simulink model "Parabolic_sim"  (R2017a)
settings: Solver=VariableStepAuto  StartTime=0.0  StopTime=50  RelTol=1e-3
values from neighbouring files (symbols this model uses):
  b = 2.8956    [Aerosonde_coeff.m]    (also in coeff_Aerosonde.m)
  c = 0.18994    [Aerosonde_coeff.m]    (also in coeff_Aerosonde.m)
  C_De = 0    [Aerosonde_coeff.m]    (also in coeff_Aerosonde.m)
  C_Dq = 0    [Aerosonde_coeff.m]    (also in coeff_Aerosonde.m)
  C_Le = -0.36    [Aerosonde_coeff.m]    (also in coeff_Aerosonde.m)
  C_Lq = 0    [Aerosonde_coeff.m]    (also in coeff_Aerosonde.m)
  C_m0 = -0.02338    [Aerosonde_coeff.m]    (also in coeff_Aerosonde.m)
  C_ma = -0.38    [Aerosonde_coeff.m]    (also in coeff_Aerosonde.m)
  C_me = -0.5    [Aerosonde_coeff.m]    (also in coeff_Aerosonde.m)
  C_mq = -3.6    [Aerosonde_coeff.m]    (also in coeff_Aerosonde.m)
  rho = 1.2682    [Aerosonde_coeff.m]    (also in coeff_Aerosonde.m)
undefined symbols (not defined in the file or in its folder): Newton, Raphson, sigbuilder_block
libraries: simulink_extras x7, aerolibasang x3, shared3dof x1, aerolibadyn x1
settings Model: Creator=jljoberg  LastModifiedBy=jljoberg

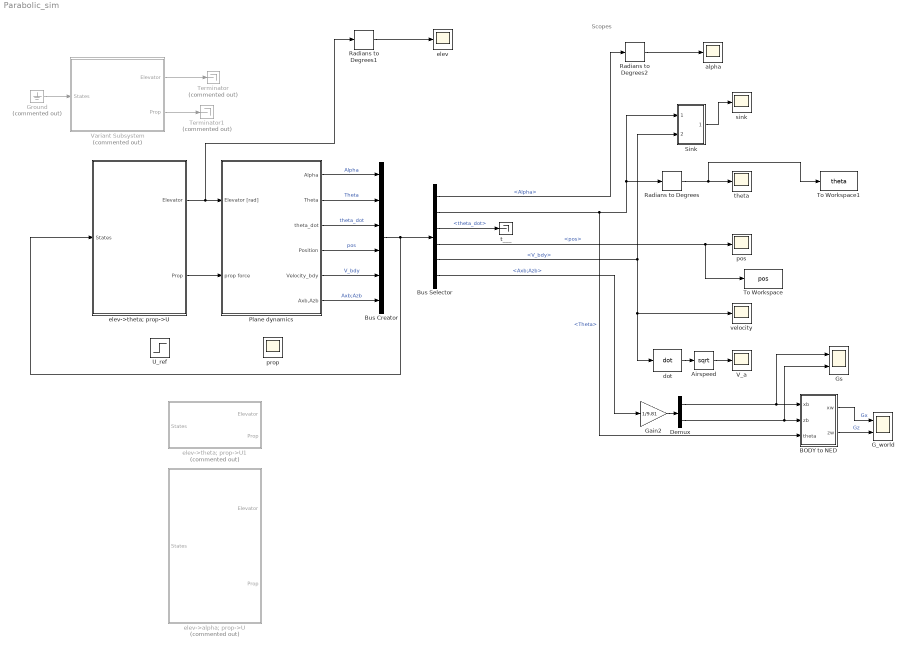
== system Parabolic_sim ==
  note: Scopes
  Airspeed : Sqrt  AlgorithmType=Newton-Raphson  SaturateOnIntegerOverflow=on
  BODY to NED : Subsystem
  Bus Creator : BusCreator  Inputs=6
  Bus Selector : BusSelector  OutputSignals=Alpha,Theta,theta_dot,pos,V_bdy,Axb;Azb
  Demux : Demux  Outputs=2
  G_world : Scope  NumInputPorts=2
  Gain2 : Gain  Gain=1/9.81
  Ground : Ground  Commented=on
  Gs : Scope  NumInputPorts=2
  Plane dynamics : Subsystem
  Radians to Degrees : simulink_extras/Transformations/Radians to Degrees
  Radians to Degrees1 : simulink_extras/Transformations/Radians to Degrees
  Radians to Degrees2 : simulink_extras/Transformations/Radians to Degrees
  Sink : Subsystem
  Terminator : Terminator  Commented=on
  Terminator1 : Terminator  Commented=on
  To Workspace : ToWorkspace  VariableName=pos  SaveFormat=Timeseries  SampleTime=-1
  To Workspace1 : ToWorkspace  VariableName=theta  SaveFormat=Timeseries  SampleTime=-1
  U_ref : Step  Time=10.5  Before=10  After=5  SampleTime=0
  V_a : Scope
  Variant Subsystem : Subsystem  Commented=on  Variant=on  OverrideUsingVariant=(default)
  alpha : Scope
  dot : aerolibasang/Incidence  & Airspeed/dot
      settings: SourceProductName=Aerospace Blockset  SourceProductBaseCode=AE
  elev : Scope
  elev->alpha; prop->U : Subsystem  Commented=on  VariantControl=Variant
  elev->theta; prop->U : Subsystem  VariantControl=Variant
  elev->theta; prop->U1 : Subsystem  Commented=on  VariantControl=(default)
  pos : Scope
  prop : Scope
  sink : Scope
  t___ : Terminator
  theta : Scope
  velocity : Scope
  wires:
  Bus Selector/1 -> Radians to Degrees2/1  "<Alpha>"
  Bus Selector/2 -> BODY to NED/3(theta), Radians to Degrees/1, Sink/1(theta)  "<Theta>"
  Bus Selector/3 -> t___/1  "<theta_dot>"
  Bus Selector/4 -> To Workspace/1, pos/1  "<pos>"
  Bus Selector/5 -> dot/1, velocity/1, Sink/2(v_bdy)  "<V_bdy>"
  Airspeed/1 -> V_a/1
  dot/1 -> Airspeed/1
  Radians to Degrees/1 -> To Workspace1/1, theta/1
  Sink/1(sink) -> sink/1
  Plane dynamics/6(Axb,Azb) -> Bus Creator/6  "Axb;Azb"
  Plane dynamics/5(Velocity_bdy) -> Bus Creator/5  "V_bdy"
  Plane dynamics/4(Position) -> Bus Creator/4  "pos"
  Plane dynamics/3(theta_dot) -> Bus Creator/3  "theta_dot"
  Plane dynamics/2(Theta) -> Bus Creator/2  "Theta"
  Plane dynamics/1(Alpha) -> Bus Creator/1  "Alpha"
  Bus Creator/1 -> elev->theta; prop->U/1(States), Bus Selector/1
  Radians to Degrees2/1 -> alpha/1
  Ground/1 -> Variant Subsystem/1(States)
  Variant Subsystem/1(Elevator) -> Terminator/1
  Variant Subsystem/2(Prop) -> Terminator1/1
  Bus Selector/6 -> Gain2/1  "<Axb;Azb>"
  Radians to Degrees1/1 -> elev/1
  elev->theta; prop->U/1(Elevator) -> Radians to Degrees1/1, Plane dynamics/1(Elevator [rad])
  Gain2/1 -> Demux/1
  Demux/1 -> BODY to NED/1(xb), Gs/1
  Demux/2 -> BODY to NED/2(zb), Gs/2
  BODY to NED/1(xw) -> G_world/1  "Gx"
  BODY to NED/2(zw) -> G_world/2  "Gz"
  elev->theta; prop->U/2(Prop) -> Plane dynamics/2(prop force)

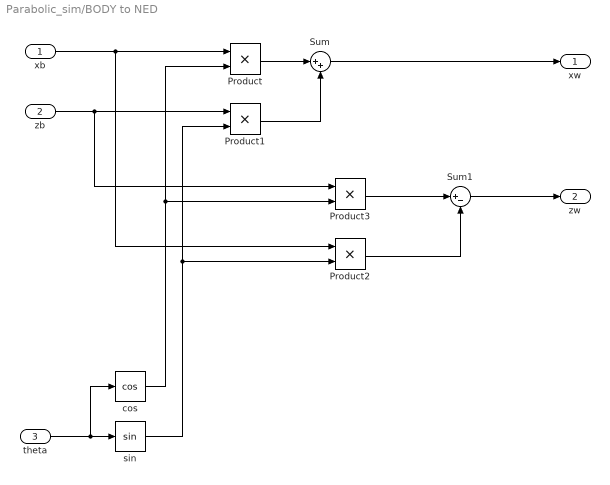
== system Parabolic_sim/BODY to NED ==
  xb : Inport
  zb : Inport  Port=2
  theta : Inport  Port=3
  Product{,1..3} (4 alike) : Product
  Sum : Sum  Inputs=|++
  Sum1 : Sum  Inputs=|+-
  "cos " : Trigonometry  Operator=cos
  sin : Trigonometry
  xw : Outport
  zw : Outport  Port=2
  wires:
  theta/1 -> sin/1, "cos "/1
  xb/1 -> Product/1, Product2/1
  "cos "/1 -> Product3/2, Product/2
  Product/1 -> Sum/1
  Sum/1 -> xw/1
  zb/1 -> Product3/1, Product1/1
  sin/1 -> Product1/2, Product2/2
  Product1/1 -> Sum/2
  Sum1/1 -> zw/1
  Product3/1 -> Sum1/1
  Product2/1 -> Sum1/2

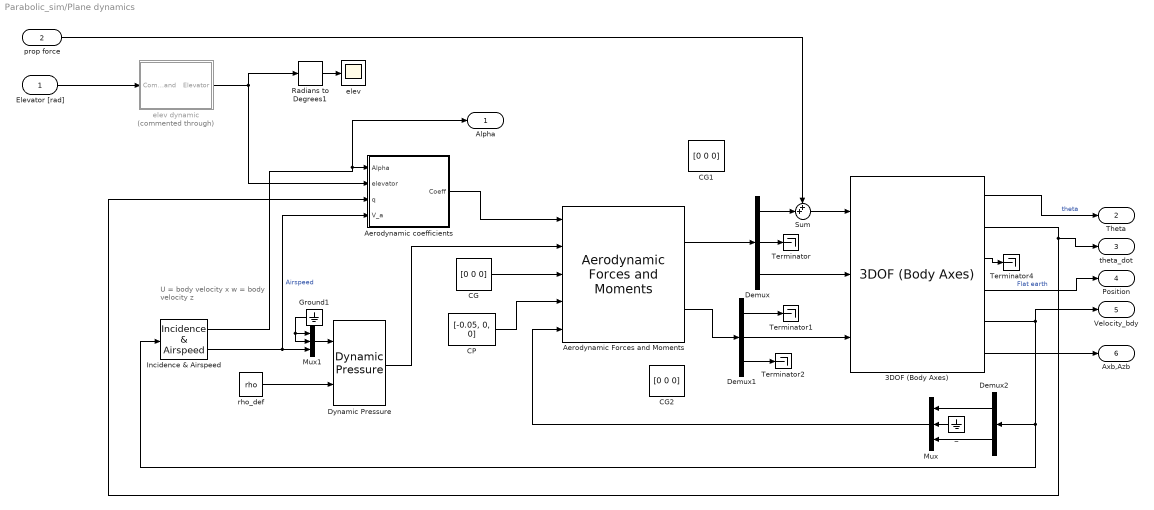
== system Parabolic_sim/Plane dynamics ==
  note: U = body velocity x
      | w = body velocity z
  Elevator [rad] : Inport
  prop force : Inport  Port=2
  3DOF (Body Axes) : shared3dof/3DOF (Body Axes)  units=Metric (MKS)  mtype=Fixed  v_ini=30  theta_ini=60*deg2rad  alpha_ini=0  q_ini=0*deg2rad  pos_ini=[0 0]  mass=m  mass_e=0.5  mass_f=3.0  Iyy=Jy  Iyy_e=0.5  Iyy_f=3.0  g_in=Internal  g=9.81  vre_flag=on  abi_flag=off
  "Aerodynamic Forces and Moments " : aerolibadyn/Aerodynamic Forces and Moments   inputAxes=Wind  outputForceAxes=Body  outputMomentAxes=Wind  S=S  b=b  cbar=1
      settings: SourceProductName=Aerospace Blockset
  Aerodynamic coefficients : Subsystem
  CG : Constant  Value=[0 0 0]
  CG1 : Constant  Value=[0 0 0]
  CG2 : Constant  Value=[0 0 0]
  CP : Constant  Value=[-0.05, 0, 0]
  Demux : Demux  Outputs=3
  Demux1 : Demux  Outputs=3
  Demux2 : Demux  Outputs=2
  Dynamic Pressure : aerolibasang/Dynamic Pressure
  Ground1 : Ground
  Incidence & Airspeed : aerolibasang/Incidence  & Airspeed
      settings: SourceProductName=Aerospace Blockset  SourceProductBaseCode=AE
  Mux : Mux  Inputs=3
  Mux1 : Mux  Inputs=3
  Radians to Degrees1 : simulink_extras/Transformations/Radians to Degrees
  Sum : Sum  Inputs=++|
  Terminator{,1..2,4} (4 alike) : Terminator
  _ : Ground
  elev : Scope
  elev dynamic : Subsystem  Commented=through
  rho_def : Constant  Value=rho
  Alpha : Outport
  Theta : Outport  Port=2
  theta_dot : Outport  Port=3
  Position : Outport  Port=4
  Velocity_bdy : Outport  Port=5
  Axb,Azb : Outport  Port=6
  wires:
  Ground1/1 -> Mux1/1, Mux1/2
  3DOF (Body Axes)/2 -> Aerodynamic coefficients/3(q), theta_dot/1
  3DOF (Body Axes)/3 -> Terminator4/1
  Incidence & Airspeed/1 -> Alpha/1, Aerodynamic coefficients/1(Alpha)
  rho_def/1 -> Dynamic Pressure/2
  Aerodynamic coefficients/1(Coeff) -> "Aerodynamic Forces and Moments "/1
  Incidence & Airspeed/2 -> Mux1/3, Aerodynamic coefficients/4(V_a)  "Airspeed"
  3DOF (Body Axes)/5 -> Velocity_bdy/1, Incidence & Airspeed/1, Demux2/1
  Dynamic Pressure/1 -> "Aerodynamic Forces and Moments "/2
  Demux/3 -> 3DOF (Body Axes)/2
  3DOF (Body Axes)/1 -> Theta/1  "theta"
  3DOF (Body Axes)/6 -> Axb,Azb/1
  Demux/2 -> Terminator/1
  3DOF (Body Axes)/4 -> Position/1  "Flat earth"
  CG/1 -> "Aerodynamic Forces and Moments "/3
  CP/1 -> "Aerodynamic Forces and Moments "/4
  Demux2/1 -> Mux/1
  Demux1/2 -> 3DOF (Body Axes)/3
  _/1 -> Mux/2
  Demux1/1 -> Terminator1/1
  Demux1/3 -> Terminator2/1
  Demux2/2 -> Mux/3
  Mux/1 -> "Aerodynamic Forces and Moments "/5
  Mux1/1 -> Dynamic Pressure/1
  Sum/1 -> 3DOF (Body Axes)/1
  prop force/1 -> Sum/1
  Demux/1 -> Sum/2
  Radians to Degrees1/1 -> elev/1
  Elevator [rad]/1 -> elev dynamic/1(Command)
  elev dynamic/1(Elevator) -> Aerodynamic coefficients/2(elevator), Radians to Degrees1/1
  "Aerodynamic Forces and Moments "/2 -> Demux1/1
  "Aerodynamic Forces and Moments "/1 -> Demux/1

== system Parabolic_sim/Sink ==
  theta : Inport
  v_bdy : Inport  Port=2
  Demux : Demux  Outputs=2
  Product : Product
  Product1 : Product
  Sum : Sum  Inputs=-+|
  Trigonometric Function : Trigonometry  Operator=cos
  Trigonometric Function1 : Trigonometry
  sink : Outport
  wires:
  v_bdy/1 -> Demux/1
  theta/1 -> Trigonometric Function1/1, Trigonometric Function/1
  Product/1 -> Sum/2
  Product1/1 -> Sum/1
  Sum/1 -> sink/1
  Trigonometric Function/1 -> Product/2
  Demux/2 -> Product/1
  Demux/1 -> Product1/2
  Trigonometric Function1/1 -> Product1/1

== system Parabolic_sim/Variant Subsystem ==
  note: 1) Add Subsystem or Model blocks as valid variant choices.
      | 2) You cannot connect blocks at this level. At simulation, connectivity is automatically
      | determined, based on the active variant and port name matching.
  States : Inport
  elev->theta; prop->U : Subsystem  VariantControl=(default)
  Elevator : Outport
  Prop : Outport  Port=2

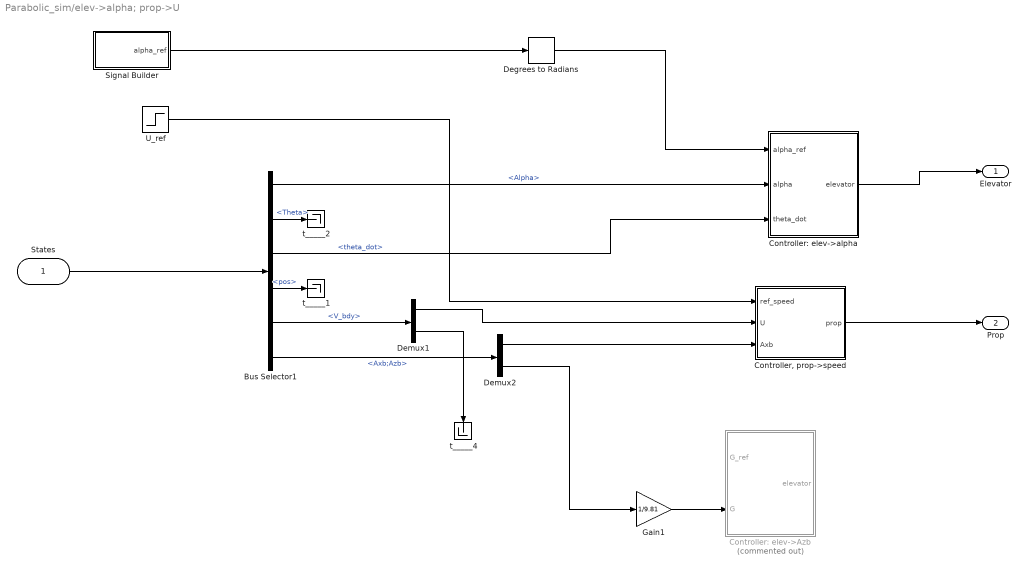
== system Parabolic_sim/elev->alpha; prop->U ==
  States : Inport
  Bus Selector1 : BusSelector  OutputSignals=Alpha,Theta,theta_dot,pos,V_bdy,Axb;Azb
  "Controller, prop->speed" : Subsystem
  Controller: elev->Azb : Subsystem  Commented=on
  Controller: elev->alpha : Subsystem
  Degrees to Radians : simulink_extras/Transformations/Degrees to Radians
  Demux1 : Demux  Outputs=2
  Demux2 : Demux  Outputs=2
  Gain1 : Gain  Gain=1/9.81
  Signal Builder : Subsystem  Tag=STV Subsys  LoadFcn=sigbuilder_block('load');  StartFcn=sigbuilder_block('start');  StopFcn=sigbuilder_block('stop');  ClipboardFcn=sigbuilder_block('clipboard');  mask(Sigbuilder block){tuvar=[0:10]}
      mask help: Simulink:masks:SigbuilderBlock_MD
      mask init:
      | if ~strcmp(get_param(bdroot(gcbh),'SimulationStatus'),'stopped') tuvar = sigbuilder_block('maskInit'); end
      settings: CopyFcn=sigbuilder_block('copy');  DeleteFcn=sigbuilder_block('delete');  ModelCloseFcn=sigbuilder_block('modelClose');  PreSaveFcn=sigbuilder_block('preSave');  PauseFcn=sigbuilder_block('pause');  ContinueFcn=sigbuilder_block('continue');  NameChangeFcn=sigbuilder_block('namechange');  OpenFcn=sigbuilder_block('open',[254.25 194.25 787.5 402 ]);  CloseFcn=sigbuilder_block('close');
      mask Display: plot(0, 0, 100, 100,[2, 2, 32, 32, 2], [68, 8, 8, 68, 68],[32, 2], [38, 38], [32, 19, 2],[53, 60, 44], [32, 17, 17, 2],[16, 16, 31, 31]);txt = getActiveGroup(gcbh);text(2, 100, txt,'verticalAlignment', 'top');
  U_ref : Step  Time=150  Before=25  After=25  SampleTime=0
  t_____1 : Terminator
  t_____2 : Terminator
  t_____4 : Terminator
  Elevator : Outport
  Prop : Outport  Port=2
  wires:
  "Controller, prop->speed"/1(prop) -> Prop/1
  Demux1/1 -> "Controller, prop->speed"/2(U)
  Demux2/2 -> Gain1/1
  Bus Selector1/5 -> Demux1/1  "<V_bdy>"
  Bus Selector1/6 -> Demux2/1  "<Axb;Azb>"
  Demux2/1 -> "Controller, prop->speed"/3(Axb)
  States/1 -> Bus Selector1/1
  Demux1/2 -> t_____4/1
  Bus Selector1/4 -> t_____1/1  "<pos>"
  Gain1/1 -> Controller: elev->Azb/2(G)
  Controller: elev->alpha/1(elevator) -> Elevator/1
  Bus Selector1/1 -> Controller: elev->alpha/2(alpha)  "<Alpha>"
  U_ref/1 -> "Controller, prop->speed"/1(ref_speed)
  Signal Builder/1(alpha_ref) -> Degrees to Radians/1
  Degrees to Radians/1 -> Controller: elev->alpha/1(alpha_ref)
  Bus Selector1/2 -> t_____2/1  "<Theta>"
  Bus Selector1/3 -> Controller: elev->alpha/3(theta_dot)  "<theta_dot>"

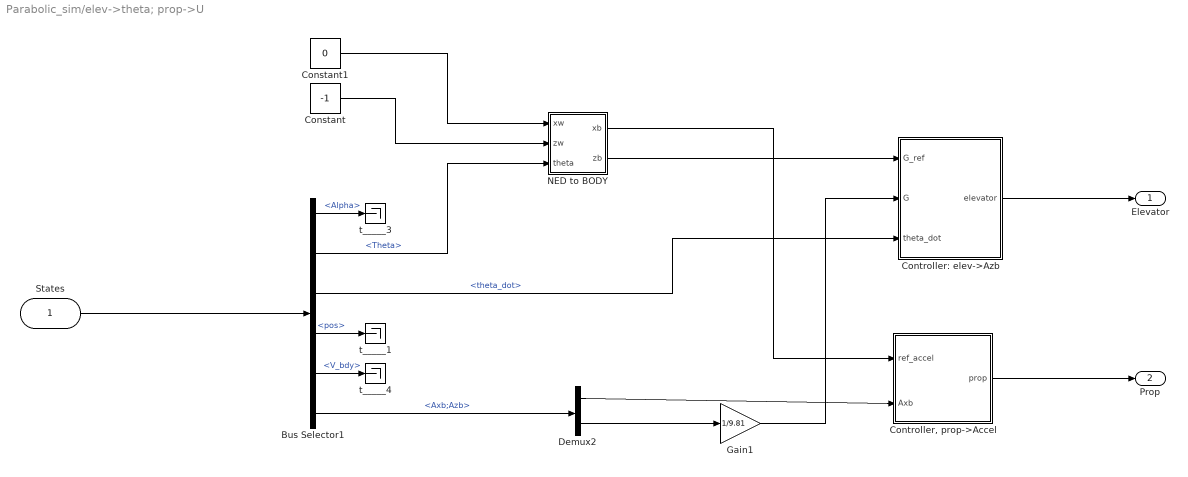
== system Parabolic_sim/elev->theta; prop->U ==
  States : Inport
  Bus Selector1 : BusSelector  OutputSignals=Alpha,Theta,theta_dot,pos,V_bdy,Axb;Azb
  Constant : Constant  Value=-1
  Constant1 : Constant  Value=0
  "Controller, prop->Accel" : Subsystem
  Controller: elev->Azb : Subsystem
  Demux2 : Demux  Outputs=2
  Gain1 : Gain  Gain=1/9.81
  NED to BODY : Subsystem
  t_____1 : Terminator
  t_____3 : Terminator
  t_____4 : Terminator
  Elevator : Outport
  Prop : Outport  Port=2
  wires:
  "Controller, prop->Accel"/1(prop) -> Prop/1
  Demux2/2 -> Gain1/1
  Bus Selector1/6 -> Demux2/1  "<Axb;Azb>"
  Demux2/1 -> "Controller, prop->Accel"/2(Axb)
  States/1 -> Bus Selector1/1
  Bus Selector1/4 -> t_____1/1  "<pos>"
  Gain1/1 -> Controller: elev->Azb/2(G)
  Controller: elev->Azb/1(elevator) -> Elevator/1
  Bus Selector1/1 -> t_____3/1  "<Alpha>"
  Bus Selector1/2 -> NED to BODY/3(theta)  "<Theta>"
  Bus Selector1/3 -> Controller: elev->Azb/3(theta_dot)  "<theta_dot>"
  Constant/1 -> NED to BODY/2(zw)
  Constant1/1 -> NED to BODY/1(xw)
  NED to BODY/2(zb) -> Controller: elev->Azb/1(G_ref)
  NED to BODY/1(xb) -> "Controller, prop->Accel"/1(ref_accel)
  Bus Selector1/5 -> t_____4/1  "<V_bdy>"

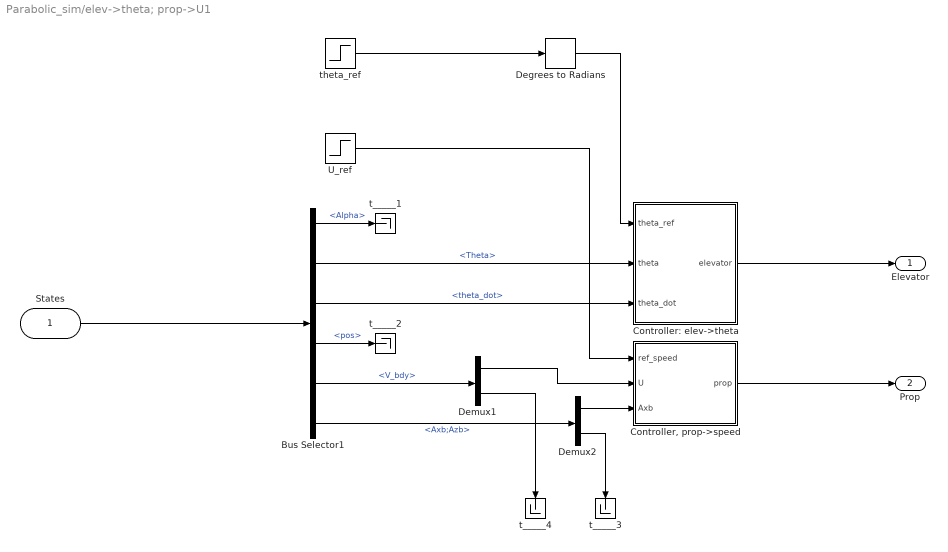
== system Parabolic_sim/elev->theta; prop->U1 ==
  States : Inport
  Bus Selector1 : BusSelector  OutputSignals=Alpha,Theta,theta_dot,pos,V_bdy,Axb;Azb
  "Controller, prop->speed" : Subsystem
  Controller: elev->theta : Subsystem
  Degrees to Radians : simulink_extras/Transformations/Degrees to Radians
  Demux1 : Demux  Outputs=2
  Demux2 : Demux  Outputs=2
  U_ref : Step  Time=150  Before=20  After=30  SampleTime=0
  t_____{1..4} (4 alike) : Terminator
  theta_ref : Step  Time=180  After=30  SampleTime=0
  Elevator : Outport
  Prop : Outport  Port=2
  wires:
  theta_ref/1 -> Degrees to Radians/1
  Degrees to Radians/1 -> Controller: elev->theta/1(theta_ref)
  Controller: elev->theta/1(elevator) -> Elevator/1
  "Controller, prop->speed"/1(prop) -> Prop/1
  Bus Selector1/2 -> Controller: elev->theta/2(theta)  "<Theta>"
  Bus Selector1/3 -> Controller: elev->theta/3(theta_dot)  "<theta_dot>"
  Demux1/1 -> "Controller, prop->speed"/2(U)
  U_ref/1 -> "Controller, prop->speed"/1(ref_speed)
  Demux2/2 -> t_____3/1
  Bus Selector1/1 -> t_____1/1  "<Alpha>"
  Bus Selector1/5 -> Demux1/1  "<V_bdy>"
  Bus Selector1/6 -> Demux2/1  "<Axb;Azb>"
  Bus Selector1/4 -> t_____2/1  "<pos>"
  Demux2/1 -> "Controller, prop->speed"/3(Axb)
  States/1 -> Bus Selector1/1
  Demux1/2 -> t_____4/1

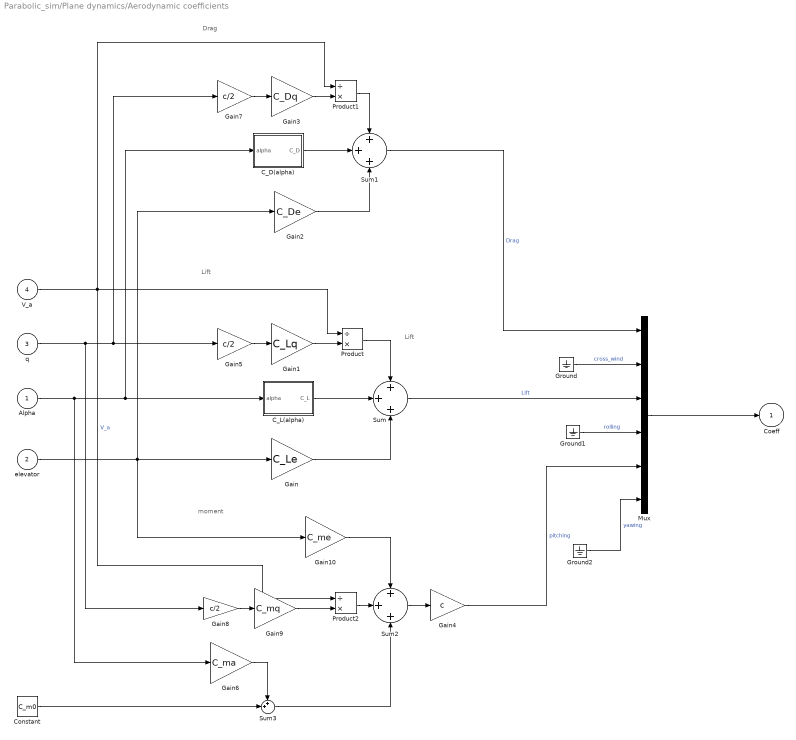
== system Parabolic_sim/Plane dynamics/Aerodynamic coefficients ==
  note: moment
  note: Lift
  note: Drag
  note: Lift
  Alpha : Inport
  elevator : Inport  Port=2
  q : Inport  Port=3
  V_a : Inport  Port=4
  C_D(alpha) : MATLAB Function  TreatAsAtomicUnit=on
  C_L(alpha) : MATLAB Function  TreatAsAtomicUnit=on
  Constant : Constant  Value=C_m0
  Gain : Gain  Gain=C_Le
  Gain1 : Gain  Gain=C_Lq
  Gain10 : Gain  Gain=C_me
  Gain2 : Gain  Gain=C_De
  Gain3 : Gain  Gain=C_Dq
  Gain4 : Gain  Gain=c
  Gain5 : Gain  Gain=c/2
  Gain6 : Gain  Gain=C_ma
  Gain7 : Gain  Gain=c/2
  Gain8 : Gain  Gain=c/2
  Gain9 : Gain  Gain=C_mq
  Ground : Ground
  Ground1 : Ground
  Ground2 : Ground
  Mux : Mux  Inputs=6
  Product : Product  Inputs=/*
  Product1 : Product  Inputs=/*
  Product2 : Product  Inputs=/*
  Sum : Sum  Inputs=+++
  Sum1 : Sum  Inputs=+++
  Sum2 : Sum  Inputs=+++
  Sum3 : Sum  Inputs=++|
  Coeff : Outport
  wires:
  Alpha/1 -> Gain6/1, C_D(alpha)/1(alpha), C_L(alpha)/1(alpha)
  C_L(alpha)/1(C_L) -> Sum/2
  Gain/1 -> Sum/3
  Sum/1 -> Mux/3  "Lift"
  Ground/1 -> Mux/2  "cross_wind"
  Ground1/1 -> Mux/4  "rolling"
  Ground2/1 -> Mux/6  "yawing"
  C_D(alpha)/1(C_D) -> Sum1/2
  Gain2/1 -> Sum1/3
  q/1 -> Gain8/1, Gain7/1, Gain5/1
  V_a/1 -> Product2/1, Product/1, Product1/1  "V_a"
  Gain1/1 -> Product/2
  Product/1 -> Sum/1
  Gain5/1 -> Gain1/1
  Gain3/1 -> Product1/2
  Product1/1 -> Sum1/1
  Gain7/1 -> Gain3/1
  Sum1/1 -> Mux/1  "Drag"
  Sum2/1 -> Gain4/1
  Gain4/1 -> Mux/5  "pitching"
  Constant/1 -> Sum3/2
  Sum3/1 -> Sum2/3
  Gain6/1 -> Sum3/1
  Product2/1 -> Sum2/2
  Gain8/1 -> Gain9/1
  Gain9/1 -> Product2/2
  Gain10/1 -> Sum2/1
  elevator/1 -> Gain10/1, Gain2/1, Gain/1
  Mux/1 -> Coeff/1

== system Parabolic_sim/Plane dynamics/elev dynamic ==
  Command : Inport
  Gain : Gain  Gain=9999
  Integrator : Integrator
  Scope : Scope
  Sum : Sum  Inputs=|+-
  Elevator : Outport
  wires:
  Integrator/1 -> Scope/1, Elevator/1, Sum/2
  Sum/1 -> Gain/1
  Gain/1 -> Integrator/1
  Command/1 -> Sum/1

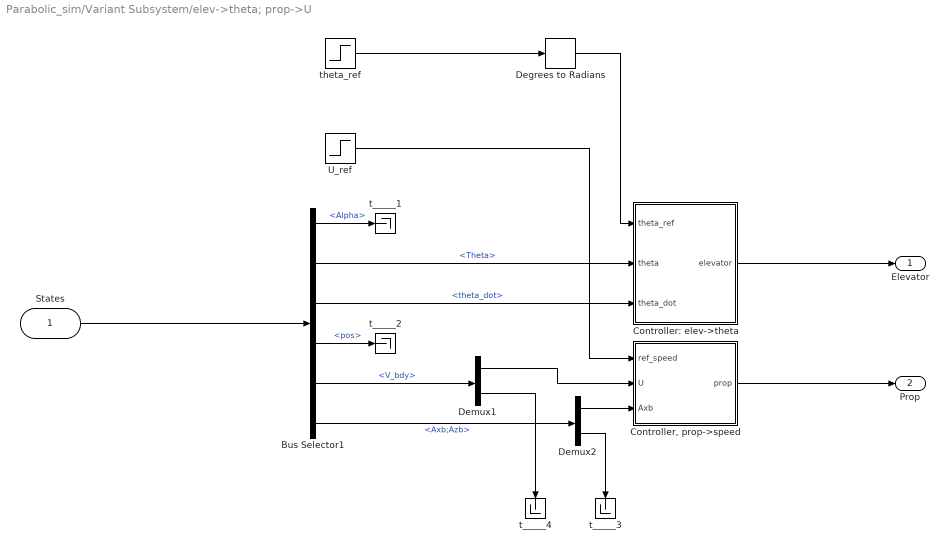
== system Parabolic_sim/Variant Subsystem/elev->theta; prop->U ==
  States : Inport
  Bus Selector1 : BusSelector  OutputSignals=Alpha,Theta,theta_dot,pos,V_bdy,Axb;Azb
  "Controller, prop->speed" : Subsystem
  Controller: elev->theta : Subsystem
  Degrees to Radians : simulink_extras/Transformations/Degrees to Radians
  Demux1 : Demux  Outputs=2
  Demux2 : Demux  Outputs=2
  U_ref : Step  Time=150  Before=20  After=30  SampleTime=0
  t_____{1..4} (4 alike) : Terminator
  theta_ref : Step  Time=180  After=60  SampleTime=0
  Elevator : Outport
  Prop : Outport  Port=2
  wires:
  theta_ref/1 -> Degrees to Radians/1
  Degrees to Radians/1 -> Controller: elev->theta/1(theta_ref)
  Controller: elev->theta/1(elevator) -> Elevator/1
  "Controller, prop->speed"/1(prop) -> Prop/1
  Bus Selector1/2 -> Controller: elev->theta/2(theta)  "<Theta>"
  Bus Selector1/3 -> Controller: elev->theta/3(theta_dot)  "<theta_dot>"
  Demux1/1 -> "Controller, prop->speed"/2(U)
  U_ref/1 -> "Controller, prop->speed"/1(ref_speed)
  Demux2/2 -> t_____3/1
  Bus Selector1/1 -> t_____1/1  "<Alpha>"
  Bus Selector1/5 -> Demux1/1  "<V_bdy>"
  Bus Selector1/6 -> Demux2/1  "<Axb;Azb>"
  Bus Selector1/4 -> t_____2/1  "<pos>"
  Demux2/1 -> "Controller, prop->speed"/3(Axb)
  States/1 -> Bus Selector1/1
  Demux1/2 -> t_____4/1

== system Parabolic_sim/elev->alpha; prop->U/Controller, prop->speed ==
  ref_speed : Inport
  U : Inport  Port=2
  Axb : Inport  Port=3
  Integrator : Integrator
  Saturation : Saturate  UpperLimit=80*1  LowerLimit=-80
  Sum : Sum  Inputs=+++
  Sum1 : Sum  Inputs=|+-
  kd : Gain  Gain=-70
  ki : Gain  Gain=0.5
  kp : Gain  Gain=20
  prop : Outport
  wires:
  Sum/1 -> Saturation/1
  kp/1 -> Sum/2
  ki/1 -> Integrator/1
  Integrator/1 -> Sum/1
  kd/1 -> Sum/3
  Axb/1 -> kd/1
  Sum1/1 -> ki/1, kp/1
  ref_speed/1 -> Sum1/1
  U/1 -> Sum1/2
  Saturation/1 -> prop/1

== system Parabolic_sim/elev->alpha; prop->U/Controller: elev->Azb ==
  G_ref : Inport
  G : Inport  Port=2
  Integrator : Integrator
  Saturation : Saturate  UpperLimit=2*pi/5  LowerLimit=-2*pi/5
  Sum : Sum  Inputs=+-|
  Sum1 : Sum  Inputs=++|
  ki : Gain  Gain=-0.5
  kp : Gain  Gain=-0.1
  elevator : Outport
  wires:
  G/1 -> Sum/2
  G_ref/1 -> Sum/1
  Sum/1 -> ki/1, kp/1
  ki/1 -> Integrator/1
  kp/1 -> Sum1/2
  Integrator/1 -> Sum1/1
  Saturation/1 -> elevator/1
  Sum1/1 -> Saturation/1

== system Parabolic_sim/elev->alpha; prop->U/Controller: elev->alpha ==
  alpha_ref : Inport
  alpha : Inport  Port=2
  theta_dot : Inport  Port=3
  Integrator : Integrator
  Saturation : Saturate  UpperLimit=2*pi/5  LowerLimit=-2*pi/5
  Sum : Sum  Inputs=+-|
  Sum1 : Sum  Inputs=+++
  "kd " : Gain
  ki : Gain  Gain=-0.3
  kp : Gain  Gain=-6
  elevator : Outport
  wires:
  Sum1/1 -> Saturation/1
  Saturation/1 -> elevator/1
  Integrator/1 -> Sum1/1
  kp/1 -> Sum1/2
  ki/1 -> Integrator/1
  Sum/1 -> kp/1, ki/1
  alpha_ref/1 -> Sum/1
  alpha/1 -> Sum/2
  theta_dot/1 -> "kd "/1
  "kd "/1 -> Sum1/3

== system Parabolic_sim/elev->alpha; prop->U/Signal Builder ==
  Demux : Demux  Tag=STV Demux  Outputs=1
  FromWs : FromWorkspace  Tag=STV FromWs  VariableName=tuvar  SampleTime=0
      SigBuilderData=|
      | common.afterFinalStr = 'Extrapolate'
      | common.sampleTime = 0
      | dataSet.timeRange = [0 600]
      | dataSet.name = 'Group 1'
      | sbobj.Groups.Name = 'Group 1'
      | sbobj.Groups.Signals.Name = 'alpha_ref'
      | sbobj.Groups.Signals.XData = [0 10 10 18.2 18.2 21.8 21.8 600]
      | sbobj.Groups.Signals.YData = [0 0 10.1 10.1 0.05 0.05 2.3 2.3]
      | sbobj.Groups.TimeRange = [0 600]
  alpha_ref : Outport  Tag=STV Outport
  wires:
  Demux/1 -> alpha_ref/1
  FromWs/1 -> Demux/1

== system Parabolic_sim/elev->theta; prop->U/Controller, prop->Accel ==
  ref_accel : Inport
  Axb : Inport  Port=2
  Integrator : Integrator
  Saturation : Saturate  UpperLimit=80*1  LowerLimit=-80
  Sum : Sum  Inputs=+++
  Sum1 : Sum  Inputs=|+-
  ki : Gain  Gain=0.5
  kp : Gain  Gain=20
  prop : Outport
  wires:
  Sum/1 -> Saturation/1
  ki/1 -> Integrator/1
  ref_accel/1 -> Sum1/1
  Saturation/1 -> prop/1
  Axb/1 -> Sum1/2
  Sum1/1 -> ki/1, kp/1
  kp/1 -> Sum/2
  Integrator/1 -> Sum/1

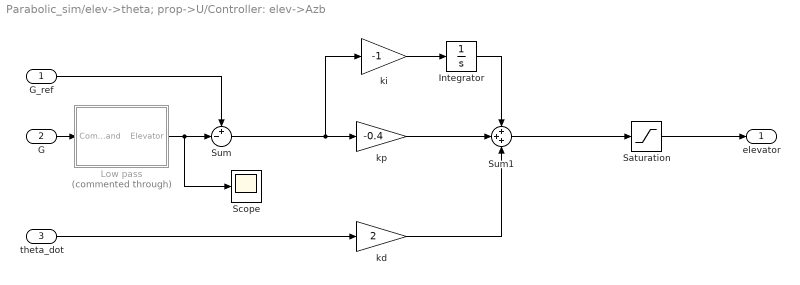
== system Parabolic_sim/elev->theta; prop->U/Controller: elev->Azb ==
  G_ref : Inport
  G : Inport  Port=2
  theta_dot : Inport  Port=3
  Integrator : Integrator  LimitOutput=on  UpperSaturationLimit=75*pi/180  LowerSaturationLimit=-75*pi/180
  Low pass : Subsystem  Commented=through
  Saturation : Saturate  UpperLimit=2*pi/5  LowerLimit=-2*pi/5
  Scope : Scope
  Sum : Sum  Inputs=+-|
  Sum1 : Sum  Inputs=+++
  kd : Gain  Gain=2
  ki : Gain  Gain=-1
  kp : Gain  Gain=-0.4
  elevator : Outport
  wires:
  G/1 -> Low pass/1(Command)
  G_ref/1 -> Sum/1
  Sum/1 -> ki/1, kp/1
  ki/1 -> Integrator/1
  kp/1 -> Sum1/2
  Integrator/1 -> Sum1/1
  Saturation/1 -> elevator/1
  Sum1/1 -> Saturation/1
  theta_dot/1 -> kd/1
  kd/1 -> Sum1/3
  Low pass/1(Elevator) -> Scope/1, Sum/2

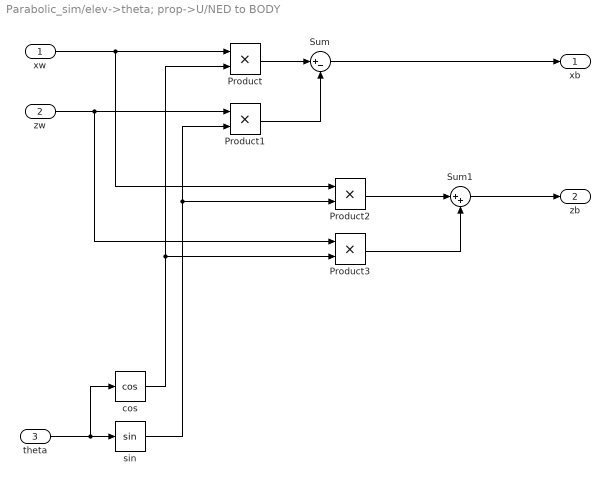
== system Parabolic_sim/elev->theta; prop->U/NED to BODY ==
  xw : Inport
  zw : Inport  Port=2
  theta : Inport  Port=3
  Product{,1..3} (4 alike) : Product
  Sum : Sum  Inputs=|+-
  Sum1 : Sum  Inputs=|++
  "cos " : Trigonometry  Operator=cos
  sin : Trigonometry
  xb : Outport
  zb : Outport  Port=2
  wires:
  theta/1 -> sin/1, "cos "/1
  xw/1 -> Product/1, Product2/1
  "cos "/1 -> Product3/2, Product/2
  Product/1 -> Sum/1
  Sum/1 -> xb/1
  zw/1 -> Product3/1, Product1/1
  sin/1 -> Product1/2, Product2/2
  Product1/1 -> Sum/2
  Product2/1 -> Sum1/1
  Product3/1 -> Sum1/2
  Sum1/1 -> zb/1

== system Parabolic_sim/elev->theta; prop->U1/Controller, prop->speed ==
  ref_speed : Inport
  U : Inport  Port=2
  Axb : Inport  Port=3
  Integrator : Integrator
  Saturation : Saturate  UpperLimit=80*1  LowerLimit=-80
  Sum : Sum  Inputs=+++
  Sum1 : Sum  Inputs=|+-
  kd : Gain  Gain=-70
  ki : Gain  Gain=0.5
  kp : Gain  Gain=20
  prop : Outport
  wires:
  Sum/1 -> Saturation/1
  kp/1 -> Sum/2
  ki/1 -> Integrator/1
  Integrator/1 -> Sum/1
  kd/1 -> Sum/3
  Axb/1 -> kd/1
  Sum1/1 -> ki/1, kp/1
  ref_speed/1 -> Sum1/1
  U/1 -> Sum1/2
  Saturation/1 -> prop/1

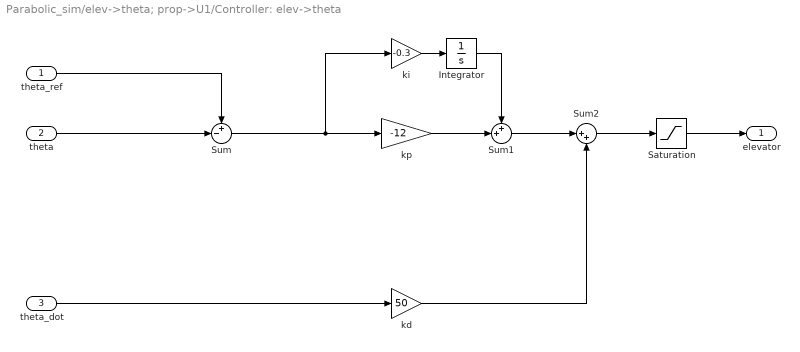
== system Parabolic_sim/elev->theta; prop->U1/Controller: elev->theta ==
  theta_ref : Inport
  theta : Inport  Port=2
  theta_dot : Inport  Port=3
  Integrator : Integrator
  Saturation : Saturate  UpperLimit=2*pi/5  LowerLimit=-2*pi/5
  Sum : Sum  Inputs=+-|
  Sum1 : Sum  Inputs=++|
  Sum2 : Sum  Inputs=|++
  kd : Gain  Gain=50
  ki : Gain  Gain=-0.3
  kp : Gain  Gain=-12
  elevator : Outport
  wires:
  theta/1 -> Sum/2
  theta_ref/1 -> Sum/1
  Sum/1 -> ki/1, kp/1
  ki/1 -> Integrator/1
  Sum1/1 -> Sum2/1
  Sum2/1 -> Saturation/1
  theta_dot/1 -> kd/1
  kd/1 -> Sum2/2
  kp/1 -> Sum1/2
  Integrator/1 -> Sum1/1
  Saturation/1 -> elevator/1

== system Parabolic_sim/Variant Subsystem/elev->theta; prop->U/Controller, prop->speed ==
  ref_speed : Inport
  U : Inport  Port=2
  Axb : Inport  Port=3
  Integrator : Integrator
  Saturation : Saturate  UpperLimit=80*1  LowerLimit=-80
  Sum : Sum  Inputs=+++
  Sum1 : Sum  Inputs=|+-
  kd : Gain  Gain=-70
  ki : Gain  Gain=0.5
  kp : Gain  Gain=20
  prop : Outport
  wires:
  Sum/1 -> Saturation/1
  kp/1 -> Sum/2
  ki/1 -> Integrator/1
  Integrator/1 -> Sum/1
  kd/1 -> Sum/3
  Axb/1 -> kd/1
  Sum1/1 -> ki/1, kp/1
  ref_speed/1 -> Sum1/1
  U/1 -> Sum1/2
  Saturation/1 -> prop/1

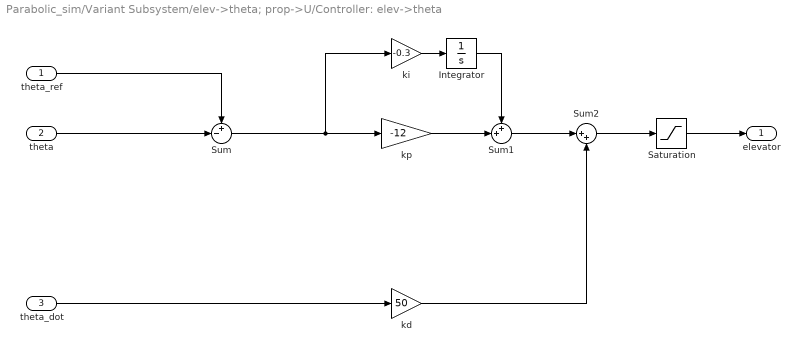
== system Parabolic_sim/Variant Subsystem/elev->theta; prop->U/Controller: elev->theta ==
  theta_ref : Inport
  theta : Inport  Port=2
  theta_dot : Inport  Port=3
  Integrator : Integrator
  Saturation : Saturate  UpperLimit=2*pi/5  LowerLimit=-2*pi/5
  Sum : Sum  Inputs=+-|
  Sum1 : Sum  Inputs=++|
  Sum2 : Sum  Inputs=|++
  kd : Gain  Gain=50
  ki : Gain  Gain=-0.3
  kp : Gain  Gain=-12
  elevator : Outport
  wires:
  theta/1 -> Sum/2
  theta_ref/1 -> Sum/1
  Sum/1 -> ki/1, kp/1
  ki/1 -> Integrator/1
  Sum1/1 -> Sum2/1
  Sum2/1 -> Saturation/1
  theta_dot/1 -> kd/1
  kd/1 -> Sum2/2
  kp/1 -> Sum1/2
  Integrator/1 -> Sum1/1
  Saturation/1 -> elevator/1

== system Parabolic_sim/elev->theta; prop->U/Controller: elev->Azb/Low pass ==
  Command : Inport
  Gain : Gain  Gain=20
  Integrator : Integrator
  Scope : Scope
  Sum : Sum  Inputs=|+-
  Elevator : Outport
  wires:
  Integrator/1 -> Scope/1, Elevator/1, Sum/2
  Sum/1 -> Gain/1
  Gain/1 -> Integrator/1
  Command/1 -> Sum/1

== matlab function Parabolic_sim/Plane dynamics/Aerodynamic coefficients/C_D(alpha) ==
  data: alpha input; C_D output
function C_D = C_D(alpha)


C_Dp    = 0.0437; 
C_L0    = 0.28;
C_La    = 3.45;
e       = 0.9;
S       = 0.55;
b       = 2.8956;
AR      = b^2/S;

C_D = C_Dp + (C_L0 + C_La*alpha)^2/(pi*e*AR);

== matlab function Parabolic_sim/Plane dynamics/Aerodynamic coefficients/C_L(alpha) ==
  data: alpha input; C_L output
function C_L = C_L(alpha)

C_L0    = 0.28; 
C_La    = 3.45;
M       = 50;

alpha_0 = 0.4712;
sigma =( 1+exp(-M*(alpha-alpha_0))+exp(M*(alpha+alpha_0)) ) ...
              / ( (1+exp(-M*(alpha-alpha_0)))*(1+exp(M*(alpha+alpha_0))) );


C_L = (1-sigma) * (C_L0 + C_La*alpha) ...
             + sigma * 2*sign(alpha)*sin(alpha)^2*cos(alpha);
